simulink subsystem "LargeMotors_ThorneFleissner"  (R2020b)
settings: Solver=VariableStepAuto  StartTime=0.0  StopTime=10.0  RelTol=1e-3
settings Model: Creator=rthom  LastModifiedBy=rthom

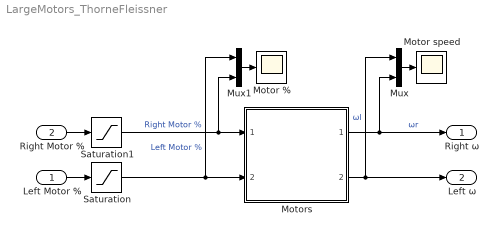
== system LargeMotors_ThorneFleissner ==
  Left Motor % : Inport
  Right Motor % : Inport  Port=2
  Motor % : Scope
  Motor speed : Scope
  Motors : Subsystem  ReferencedSubsystem=Motors_ThorneFleissner
  Mux : Mux  Inputs=2
  Mux1 : Mux  Inputs=2
  Saturation : Saturate  UpperLimit=100  LowerLimit=-100
  Saturation1 : Saturate  UpperLimit=100  LowerLimit=-100
  Right ω : Outport
  Left ω : Outport  Port=2
  wires:
  Motors/1 -> Right ω/1, Mux/2  "ωr"
  Motors/2 -> Left ω/1, Mux/1  "ωl"
  Mux/1 -> Motor speed/1
  Mux1/1 -> Motor %/1
  Saturation1/1 -> Mux1/2, Motors/1  "Right Motor %"
  Saturation/1 -> Mux1/1, Motors/2  "Left Motor %"
  Left Motor %/1 -> Saturation/1
  Right Motor %/1 -> Saturation1/1
